simulink model "ex_ip_servo"  (R2023a)
settings: Solver=ode1  StartTime=0.0  StopTime=inf  FixedStep=h  RelTol=1e-3  EnableMultiTasking=on
values from neighbouring files (symbols this model uses):
  delta1 = 1.51e+00    (= 1.51)    [ip_servo_design.m]
  G = Ke(5)    [ip_servo_design.m]
  K = Ke(1:4)    [ip_servo_design.m]
  Tf1 = 0.05    [ip_servo_design.m]
  Tf2 = 0.05    [ip_servo_design.m]
libraries: roller485lib x3, carterlib x1
settings Model: ExtModeTrigDuration=2  Creator=kawata  LastModifiedBy=kawata
settings SolverCC: AutoInsertRateTranBlk=on
settings DataIOCC: ReturnWorkspaceOutputs=off
settings OptimizationCC: EnhancedBackFolding=on  PassReuseOutputArgsThreshold=0  MaxStackSize=64  OptimizeBlockOrder=speed  DifferentSizesBufferReuse=on  OptimizationCustomize=off
settings DebuggingCC: ParameterTunabilityLossMsg=error
settings HardwareCC: ProdBitPerInt=16  ProdBitPerPointer=16  ProdBitPerSizeT=16  ProdBitPerPtrDiffT=16  ProdLargestAtomicFloat=None  ProdWordSize=8  ProdHWDeviceType=Atmel->AVR
settings SFSimCC: MATLABDynamicMemAlloc=off
settings RTWCC: Description=Embedded Coder  SystemTargetFile=ert.tlc  HardwareBoard=Arduino Mega 2560  TemplateMakefile=ert_default_tmf  Toolchain=Arduino AVR  BuildConfiguration=Faster Runs
settings CodeAppCC: ForceParamTrailComments=on  OperatorAnnotations=on
settings ERTTargetCC: ERTCustomFileBanners=off  SupportContinuousTime=on  SupportNonInlinedSFcns=on  RemoveResetFunc=off  SupportVariableSizeSignals=on  ModelStepFunctionPrototypeControlCompliant=off  ExtModeTransport=3  ExtModeStaticAlloc=on  ExtModeAutomaticAllocSize=off  ExtModeStaticAllocSize=2048  ExtModeMexFile=ext_xcp  ExtModeIntrfLevel=Level2 - Open

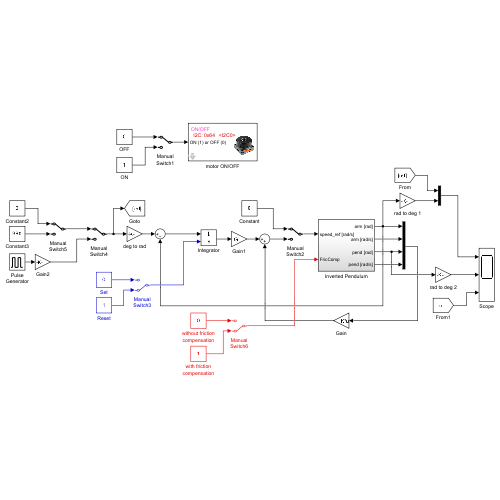
[thumbnail: Simulink's stored preview of the top-level diagram]
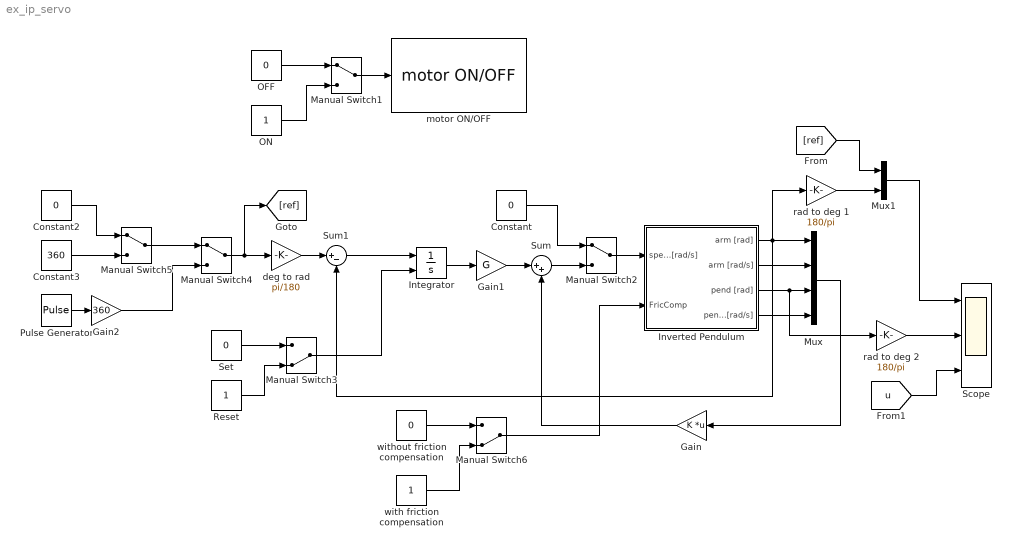
== system ex_ip_servo ==
  Constant : Constant  Value=0
  Constant2 : Constant  Value=0
  Constant3 : Constant  Value=360
  Gain : Gain  Gain=K  Multiplication=Matrix(K*u)
  Gain1 : Gain  Gain=G
  Gain2 : Gain  Gain=360
  Integrator : Integrator  ExternalReset=level hold
  Inverted Pendulum : Subsystem
  Manual Switch{1..2,4..5} (4 alike) : ManualSwitch
  Manual Switch3 : ManualSwitch  CurrentSetting=0
  Manual Switch6 : ManualSwitch  CurrentSetting=0
  Mux : Mux
  Mux1 : Mux  Inputs=2
  OFF : Constant  Value=0
  ON : Constant
  Pulse Generator : DiscretePulseGenerator  PulseType=Time based  Period=16  PulseWidth=50  PhaseDelay=4
  Reset : Constant
  Scope : Scope  NumInputPorts=3
  Set : Constant  Value=0
  Sum : Sum  Inputs=|++
  Sum1 : Sum  Inputs=|+-
  deg to rad : Gain  Gain=pi/180
  motor ON/OFF : roller485lib/motor ON//OFF  I2CAddress=0x64  I2CModule=0
      settings: SourceProductName=Roller485 Library
  rad to deg 1 : Gain  Gain=180/pi
  rad to deg 2 : Gain  Gain=180/pi
  with friction compensation : Constant
  without friction compensation : Constant  Value=0
  wires:
  Manual Switch2/1 -> Inverted Pendulum/1(speed_ref [rad/s])
  Constant/1 -> Manual Switch2/1
  Inverted Pendulum/1(arm [rad]) -> Mux/1, rad to deg 1/1, Sum1/2
  Inverted Pendulum/2(arm [rad/s]) -> Mux/2
  Inverted Pendulum/3(pend [rad]) -> Mux/3, rad to deg 2/1
  Inverted Pendulum/4(pend [rad/s]) -> Mux/4
  Mux/1 -> Gain/1
  rad to deg 2/1 -> Scope/2
  Manual Switch1/1 -> motor ON/OFF/1
  OFF/1 -> Manual Switch1/1
  ON/1 -> Manual Switch1/2
  Sum/1 -> Manual Switch2/2
  Gain/1 -> Sum/2
  Gain1/1 -> Sum/1
  Integrator/1 -> Gain1/1
  Manual Switch4/1 -> [ref], deg to rad/1
  deg to rad/1 -> Sum1/1
  Set/1 -> Manual Switch3/1
  Reset/1 -> Manual Switch3/2
  Manual Switch3/1 -> Integrator/2
  Sum1/1 -> Integrator/1
  Pulse Generator/1 -> Gain2/1
  Manual Switch5/1 -> Manual Switch4/1
  Constant2/1 -> Manual Switch5/1
  Constant3/1 -> Manual Switch5/2
  Gain2/1 -> Manual Switch4/2
  with friction compensation/1 -> Manual Switch6/2
  without friction compensation/1 -> Manual Switch6/1
  Manual Switch6/1 -> Inverted Pendulum/2(FricComp)
  rad to deg 1/1 -> Mux1/2
  [ref] -> Mux1/1
  Mux1/1 -> Scope/1
  [u] -> Scope/3

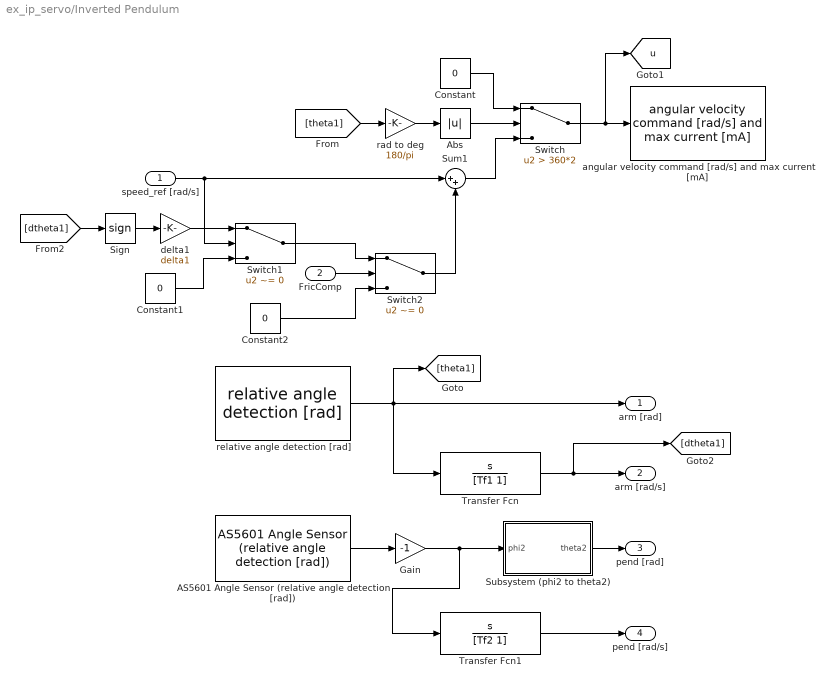
== system ex_ip_servo/Inverted Pendulum ==
  speed_ref [rad/s] : Inport
  FricComp : Inport  Port=2
  AS5601 Angle Sensor (relative angle detection [rad]) : carterlib/AS5601 Angle Sensor (relative angle detection [rad])  sample_time=-1  I2CModule=0
  Abs : Abs
  Constant : Constant  Value=0
  Constant1 : Constant  Value=0
  Constant2 : Constant  Value=0
  Gain : Gain  Gain=-1
  Sign : Signum
  Subsystem (phi2 to theta2) : Subsystem
  Sum1 : Sum  Inputs=|++
  Switch : Switch  Criteria=u2 > Threshold  Threshold=360*2  SaturateOnIntegerOverflow=off  InputSameDT=off
  Switch1 : Switch  Criteria=u2 ~= 0  SaturateOnIntegerOverflow=off  InputSameDT=off
  Switch2 : Switch  Criteria=u2 ~= 0  SaturateOnIntegerOverflow=off  InputSameDT=off
  Transfer Fcn : TransferFcn  Numerator=[1 0]  Denominator=[Tf1 1]
  Transfer Fcn1 : TransferFcn  Numerator=[1 0]  Denominator=[Tf2 1]
  angular velocity command [rad/s] and max current [mA] : roller485lib/I2C Write/angular velocity command [rad//s] and max current [mA]  I2CAddress=0x64  I2CModule=0  speed_P=2  speed_I=0  speed_D=850  max_current=1200  set_time1=0  set_time2=0  set_time3=0
      settings: SourceProductName=Roller485 Library
  delta1 : Gain  Gain=delta1
  rad to deg : Gain  Gain=180/pi
  relative angle detection [rad] : roller485lib/I2C Read/relative angle detection [rad]  I2CAddress=0x64  I2CModule=0  sample_time=-1  set_time=0
      settings: SourceProductName=Roller485 Library
  arm [rad] : Outport
  arm [rad/s] : Outport  Port=2
  pend [rad] : Outport  Port=3
  pend [rad/s] : Outport  Port=4
  tag scope: u=global
  wires:
  relative angle detection [rad]/1 -> Transfer Fcn/1, [theta1], arm [rad]/1
  Transfer Fcn/1 -> arm [rad/s]/1, [dtheta1]
  AS5601 Angle Sensor (relative angle detection [rad])/1 -> Gain/1
  Subsystem (phi2 to theta2)/1(theta2) -> pend [rad]/1
  [theta1] -> rad to deg/1
  Abs/1 -> Switch/2
  Constant/1 -> Switch/1
  rad to deg/1 -> Abs/1
  Switch/1 -> angular velocity command [rad/s] and max current [mA]/1, [u]
  Sum1/1 -> Switch/3
  speed_ref [rad/s]/1 -> Switch1/2, Sum1/1
  Constant1/1 -> Switch1/3
  delta1/1 -> Switch1/1
  [dtheta1] -> Sign/1
  Sign/1 -> delta1/1
  Gain/1 -> Transfer Fcn1/1, Subsystem (phi2 to theta2)/1(phi2)
  Switch2/1 -> Sum1/2
  FricComp/1 -> Switch2/2
  Switch1/1 -> Switch2/1
  Constant2/1 -> Switch2/3
  Transfer Fcn1/1 -> pend [rad/s]/1

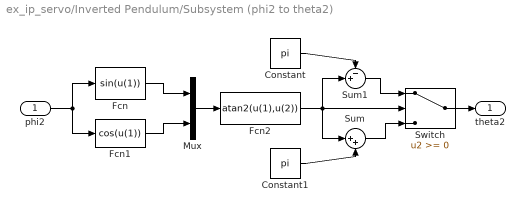
== system ex_ip_servo/Inverted Pendulum/Subsystem (phi2 to theta2) ==
  phi2 : Inport
  Constant : Constant  Value=pi
  Constant1 : Constant  Value=pi
  Fcn : Fcn  Expr=sin(u(1))
  Fcn1 : Fcn  Expr=cos(u(1))
  Fcn2 : Fcn  Expr=atan2(u(1),u(2))
  Mux : Mux  Inputs=2
  Sum : Sum  Inputs=|++  InputSameDT=on  SaturateOnIntegerOverflow=on  OutDataTypeStr=Inherit: Same as first input
  Sum1 : Sum  Inputs=-+|  InputSameDT=on  SaturateOnIntegerOverflow=on  OutDataTypeStr=Inherit: Same as first input
  Switch : Switch  SaturateOnIntegerOverflow=off  InputSameDT=off
  theta2 : Outport  VectorParamsAs1DForOutWhenUnconnected=off
  wires:
  Switch/1 -> theta2/1
  Constant/1 -> Sum1/1
  Sum/1 -> Switch/3
  Constant1/1 -> Sum/2
  Sum1/1 -> Switch/1
  Fcn2/1 -> Sum1/2, Switch/2, Sum/1
  phi2/1 -> Fcn1/1, Fcn/1
  Fcn/1 -> Mux/1
  Fcn1/1 -> Mux/2
  Mux/1 -> Fcn2/1
